simulink model "QArm_Workspace"  (R2022b)
settings: Solver=ode4  StartTime=0.0  StopTime=inf  FixedStep=1/1000  RelTol=1e-3  EnableMultiTasking=on
model workspace (MAT data in the model file):
  cameraStepSize = Simulink.Parameter
  cameraStepSize.Value = Simulink.data.Expression
  cameraStepSize.Value.ExpressionString = "qc_get_step_size * ceil (1/30 /qc_get_step_size)"
  cameraStepSize.DataType = 'auto'
  cameraStepSize.Complexity = 'real'
  cameraStepSize.Dimensions = -1
  mainStepSize = Simulink.Parameter
  mainStepSize.Value = Simulink.data.Expression
  mainStepSize.Value.ExpressionString = "qc_get_step_size"
  mainStepSize.DataType = 'auto'
  mainStepSize.Complexity = 'real'
  mainStepSize.Dimensions = -1
undefined symbols (not defined in the file or in its folder): interleaved, RGB
libraries: quarc_library x14, simulink x2
(part 1 of 2)
settings Model: SimulationMode=external  ExtModeTrigDuration=10000  Creator=mbohra  LastModifiedBy=mbohra
settings SolverCC: AlgebraicLoopSolver=TrustRegion  PositivePriorityOrder=on
settings DataIOCC: ReturnWorkspaceOutputs=off
settings DebuggingCC: UnconnectedInputMsg=warning  UnconnectedOutputMsg=warning  UnconnectedLineMsg=warning  SFMachineParentedDataDiag=warning  ArithmeticOperatorsInVariantConditions=warning
settings ModelReferenceCC: EnableRefExpFcnMdlSchedulingChecks=on
settings SFSimCC: SimUseLocalCustomCode=off  CustomCodeUndefinedFunction=UseInterfaceOnly
settings RTWCC: Description=QUARC Win64 Target Using Toolchain  SystemTargetFile=quarc_win64.tlc  TemplateMakefile=quarc_default_tmf  RTWUseLocalCustomCode=off  Toolchain=QUARC win64 | nmake (64-bit Windows)  BuildConfiguration=Faster Runs  DLArmComputeVersion=19.05
settings CodeAppCC: StateflowObjectComments=on
settings STFCustomTargetCC: TargetLangStandard=C99 (ISO)  ConcurrentExecutionCompliant=on  GRTInterface=on  UseToolchainInfoCompliant=on  SystemTargetFile=quarc_win64.tlc
settings GRTTargetCC: ParMdlRefBuildCompliant=off  CompOptLevelCompliant=off  CombineOutputUpdateFcns=off  MatFileLogging=off  CPPClassGenCompliant=off  GRTInterface=on  ExtMode=on  ExtModeMexFile=quarc_comm
settings ConfigComp: CovMetricSettings=dswe

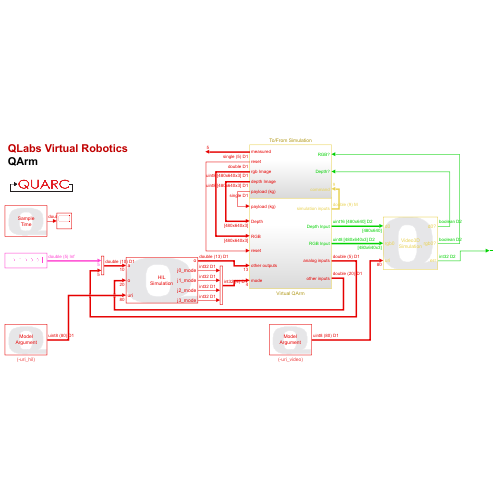
[thumbnail: Simulink's stored preview of the top-level diagram]
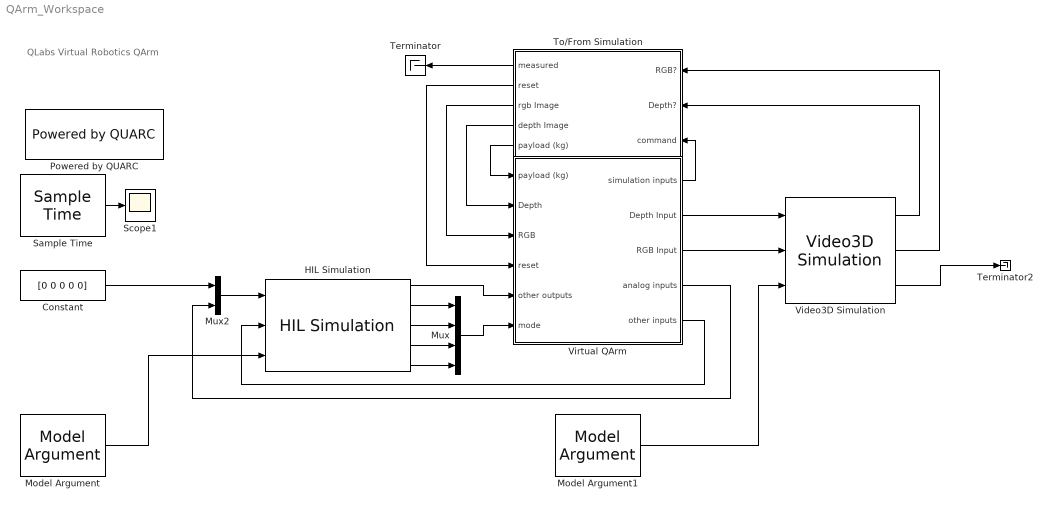
== system QArm_Workspace ==
  note: QLabs Virtual Robotics
      | QArm
  Constant : Constant  Value=[0 0 0 0 0]
  HIL Simulation : quarc_library/Data Acquisition/Generic/Configuration/HIL Simulation  uri_source=External input port  uri=tcpip://localhost:18900  board_type=qarm_usb  board_id=0  options=j0_mode=%d;j1_mode=%d;j2_mode=%d;j3_mode=%d  sample_time=qc_get_step_size  active=on  num_clocks=1  num_interrupts=0  num_analog_inputs=10  num_analog_outputs=0  initial_analog=[]  num_digital_io=0  num_digital_inputs=0  num_digital_outputs=0  initial_digital=[]  num_encoder_inputs=0  num_pwm_outputs=0  initial_pwm=[]  other_inputs=[1000:1004, 3000:3004, 10000:10004, 11000:11004]  other_outputs=[1000:1004, 11000:11003, 11005:11007, 11008]  initial_other=[0 0 0 0 0 0 0 0 0 1 0 0 1]  integer_get_property_codes=[]  double_get_property_codes=[]  string_get_property_codes=[]  integer_set_property_codes=[]  double_set_property_codes=[]  string_set_property_codes=[]  initial_integer_properties=0  initial_double_properties=0  max_string_property=80  use_variable_size_strings=off
      settings: SourceProductName=QUARC Targets
  Model Argument : quarc_library/Sources/Signals/Model Argument  argument_name=uri_hil  has_value=on  data_type_mode=Specify via dialog  data_type=char  max_length=80  default_value=0  default_string=tcpip://localhost:18900  variable_size=off
      settings: AttributesFormatString=(-%<argument_name>)  SourceProductName=QUARC Targets
  Model Argument1 : quarc_library/Sources/Signals/Model Argument  argument_name=uri_video  has_value=on  data_type_mode=Specify via dialog  data_type=char  max_length=80  default_value=0  default_string=tcpip://localhost:18901  variable_size=off
      settings: AttributesFormatString=(-%<argument_name>)  SourceProductName=QUARC Targets
  Mux : Mux
  Mux2 : Mux  Inputs=2
  Powered by QUARC : quarc_library/Logos/Powered by QUARC
  Sample Time : quarc_library/Sources/Time/Sample Time  Priority=-99  sample_time=qc_get_step_size
  Scope1 : Scope
  Terminator : Terminator
  Terminator2 : Terminator
  To/From Simulation : Subsystem
  Video3D Simulation : quarc_library/Multimedia/Video3D Simulation  uri_source=External input port  uri=tcpip://localhost:18901  device_id=0  sample_time=cameraStepSize  show_in_use=on  active=on  depth_indices=[0]  depth_scales=9.44  depth_widths=[640]  depth_heights=[480]  depth_rates=[30]  rgb_indices=[0]  rgb_widths=[640]  rgb_heights=[480]  rgb_rates=[30]  infrared_indices=[]  infrared_widths=[640]  infrared_heights=[480]  infrared_rates=[30]  fisheye_indices=[]  fisheye_widths=[640]  fisheye_heights=[480]  fisheye_rates=[30]  gyro_indices=[]  accel_indices=[]  pose_indices=[]
      settings: SourceProductName=QUARC Targets
  Virtual QArm : Subsystem
  wires:
  Mux2/1 -> HIL Simulation/1
  Constant/1 -> Mux2/1
  HIL Simulation/1 -> Virtual QArm/5(other outputs)
  Virtual QArm/4(analog inputs) -> Mux2/2
  Virtual QArm/5(other inputs) -> HIL Simulation/2
  Virtual QArm/1(simulation inputs) -> To/From Simulation/3(command)
  To/From Simulation/2(reset) -> Virtual QArm/4(reset)
  Sample Time/1 -> Scope1/1
  HIL Simulation/2 -> Mux/1
  HIL Simulation/3 -> Mux/2
  HIL Simulation/4 -> Mux/3
  HIL Simulation/5 -> Mux/4
  Mux/1 -> Virtual QArm/6(mode)
  To/From Simulation/1(measured) -> Terminator/1
  To/From Simulation/4(depth Image) -> Virtual QArm/2("Depth ")
  To/From Simulation/3(rgb Image) -> Virtual QArm/3(RGB)
  Virtual QArm/2(Depth Input) -> Video3D Simulation/1
  Virtual QArm/3(RGB Input) -> Video3D Simulation/2
  Video3D Simulation/3 -> Terminator2/1
  Video3D Simulation/1 -> To/From Simulation/2(Depth?)
  Video3D Simulation/2 -> To/From Simulation/1(RGB?)
  To/From Simulation/5(payload (kg)) -> Virtual QArm/1(payload (kg))
  Model Argument/1 -> HIL Simulation/3
  Model Argument1/1 -> Video3D Simulation/3

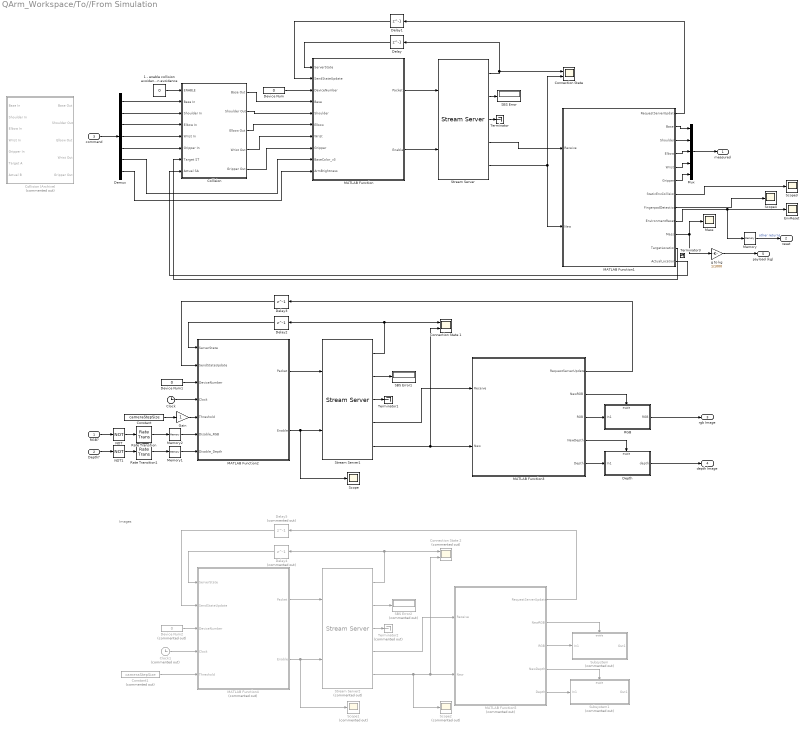
== system QArm_Workspace/To//From Simulation ==
  note: Images
  RGB? : Inport
  Depth? : Inport  Port=2
  command : Inport  Port=3
  1 - enable collision avoidance 0 - disable collision avoidance : Constant  Value=0
  Clock : Clock
  Clock1 : Clock  Commented=on
  Collision : Subsystem
  Collision (Archive) : Subsystem  Commented=on
  "Connection State " : Scope  NumInputPorts=2
  Connection State 1 : Scope  NumInputPorts=2
  Connection State 2 : Scope  Commented=on  NumInputPorts=2
  Constant : Constant  Value=cameraStepSize
  Constant1 : Constant  Commented=on  Value=cameraStepSize
  Delay : Delay  DelayLength=1
  Delay1 : Delay  DelayLength=1
  Delay2 : Delay  DelayLength=1  SampleTime=mainStepSize
  Delay3 : Delay  DelayLength=1  SampleTime=mainStepSize
  Delay4 : Delay  Commented=on  DelayLength=1  SampleTime=mainStepSize
  Delay5 : Delay  Commented=on  DelayLength=1  SampleTime=mainStepSize
  Demux : Demux  Outputs=[1 1 1 1 1 3 1 ]
  Depth : Subsystem
  Device Num : Constant  Value=0
  Device Num1 : Constant  Value=0  SampleTime=mainStepSize
  Device Num2 : Constant  Commented=on  Value=0  SampleTime=mainStepSize
  "EnvReset " : Scope
  Gain : Gain
  MATLAB Function : MATLAB Function  TreatAsAtomicUnit=on
  MATLAB Function1 : MATLAB Function  TreatAsAtomicUnit=on
  MATLAB Function2 : MATLAB Function  TreatAsAtomicUnit=on
  MATLAB Function3 : MATLAB Function  TreatAsAtomicUnit=on
  MATLAB Function4 : MATLAB Function  Commented=on  TreatAsAtomicUnit=on
  MATLAB Function5 : MATLAB Function  Commented=on  TreatAsAtomicUnit=on
  Mass : Scope
  Memory : Memory
  Memory1 : Memory
  Memory2 : Memory
  Mux : Mux  Inputs=5
  NOT : Logic  Operator=NOT  IconShape=distinctive  AllPortsSameDT=off  OutDataTypeStr=boolean
  NOT1 : Logic  Operator=NOT  IconShape=distinctive  AllPortsSameDT=off  OutDataTypeStr=boolean
  RGB : Subsystem
  Rate Transition : RateTransition
  Rate Transition1 : RateTransition
  SBS Error : Display
  SBS Error1 : Display
  SBS Error2 : Display  Commented=on
  Scope : Scope
  Scope1 : Scope  Commented=on
  Scope2 : Scope  Commented=on
  Scope3 : Scope
  Scope4 : Scope
  Stream Server : quarc_library/Communications/Basic/Stream Server  uri_source=Specify via dialog (do not evaluate)  uri=tcpip://remotehost:18001?nagle='off'  send_buffer_size=65537  receive_buffer_size=65537  byte_order=little endian (Intel - LSB first)  optimization=Minimum latency  send_options=Send all data  receive_options=Receive all data  default_value=[0]  sample_time=qc_get_step_size  active=on  implementation=Use blocking I/O in a separate thread  send_fifo_size=3  receive_fifo_size=3  send_priority=0  receive_priority=0  send_dimensions=on  receive_dimensions=on  max_dimensions=65537  data_type=uint8  type_expr=BusObject
      settings: AttributesFormatString="\"tcpip://remotehost:18001?nagle='off'\""
  Stream Server1 : quarc_library/Communications/Basic/Stream Server  uri_source=Specify via dialog (do not evaluate)  uri=tcpip://remotehost:18002?nagle='off'  send_buffer_size=65537  receive_buffer_size=100000  byte_order=little endian (Intel - LSB first)  optimization=Minimum latency  send_options=Send all data  receive_options=Receive all data  default_value=[0]  sample_time=mainStepSize  active=on  implementation=Use blocking I/O in a separate thread  send_fifo_size=3  receive_fifo_size=1  send_priority=0  receive_priority=0  send_dimensions=on  receive_dimensions=on  max_dimensions=65537  data_type=uint8  type_expr=BusObject
      settings: AttributesFormatString="\"tcpip://remotehost:18002?nagle='off'\""
  Stream Server2 : quarc_library/Communications/Basic/Stream Server  Commented=on  uri_source=Specify via dialog (do not evaluate)  uri=tcpip://remotehost:18002?nagle='off'  send_buffer_size=65537  receive_buffer_size=6000000  byte_order=little endian (Intel - LSB first)  optimization=Minimum latency  send_options=Send all data  receive_options=Receive all data  default_value=[0]  sample_time=mainStepSize  active=on  implementation=Use blocking I/O in a separate thread  send_fifo_size=3  receive_fifo_size=1  send_priority=0  receive_priority=0  send_dimensions=on  receive_dimensions=on  max_dimensions=6000000  data_type=uint8  type_expr=BusObject
      settings: AttributesFormatString="\"tcpip://remotehost:18002?nagle='off'\""
  Subsystem : Subsystem  Commented=on
  Subsystem1 : Subsystem  Commented=on
  Terminator : Terminator
  Terminator1 : Terminator
  Terminator2 : Terminator  Commented=on
  Terminator3 : Terminator
  g to kg : Gain  Gain=1/1000
  measured : Outport  VectorParamsAs1DForOutWhenUnconnected=off
  reset : Outport  Port=2  VectorParamsAs1DForOutWhenUnconnected=off
  rgb Image : Outport  Port=3
  depth Image : Outport  Port=4
  payload (kg) : Outport  Port=5
  wires:
  MATLAB Function1/1(RequestServerUpdate) -> Delay1/1
  Mux/1 -> measured/1
  Stream Server/1 -> Delay/1, "Connection State "/1
  Delay1/1 -> MATLAB Function/2(SendStateUpdate)
  Demux/7 -> MATLAB Function/10(ArmBrightness)
  MATLAB Function1/8(FingerpadDetection) -> Scope4/1
  Stream Server/3 -> Terminator/1
  MATLAB Function1/7(StaticEnvCollision) -> Scope3/1
  command/1 -> Demux/1
  Stream Server/2 -> SBS Error/1
  MATLAB Function1/3(Shoulder) -> Mux/2
  Stream Server/5 -> "Connection State "/2, MATLAB Function1/2(New)
  MATLAB Function1/10(Mass) -> Mass/1, g to kg/1
  MATLAB Function/2(Enable) -> Stream Server/2
  Device Num/1 -> MATLAB Function/3(DeviceNumber)
  MATLAB Function/1(Packet) -> Stream Server/1
  Stream Server/4 -> MATLAB Function1/1(Receive)
  MATLAB Function1/6(Gripper) -> Mux/5
  Delay/1 -> MATLAB Function/1(ServerState)
  MATLAB Function1/5(Wrist) -> Mux/4
  MATLAB Function1/4(Elbow) -> Mux/3
  MATLAB Function1/2(Base) -> Mux/1
  Demux/6 -> MATLAB Function/9(BaseColor_v3)
  MATLAB Function1/9(EnvironmentReset) -> Memory/1, "EnvReset "/1
  Memory/1 -> reset/1  "other returns"
  Stream Server1/2 -> SBS Error1/1
  MATLAB Function2/2(Enable) -> Scope/1, Stream Server1/2
  Stream Server1/1 -> Connection State 1/1, Delay2/1
  Clock/1 -> MATLAB Function2/4(Clock)
  MATLAB Function2/1(Packet) -> Stream Server1/1
  Delay2/1 -> MATLAB Function2/1(ServerState)
  Stream Server1/5 -> Connection State 1/2, MATLAB Function3/2(New)
  Stream Server1/3 -> Terminator1/1
  Device Num1/1 -> MATLAB Function2/3(DeviceNumber)
  Delay3/1 -> MATLAB Function2/2(SendStateUpdate)
  Constant/1 -> Gain/1
  Clock1/1 -> MATLAB Function4/4(Clock)
  Delay5/1 -> MATLAB Function4/2(SendStateUpdate)
  Stream Server2/2 -> SBS Error2/1
  MATLAB Function5/1(RequestServerUpdate) -> Delay5/1
  Stream Server2/3 -> Terminator2/1
  Stream Server2/5 -> Scope2/1, Connection State 2/2, MATLAB Function5/2(New)
  MATLAB Function4/1(Packet) -> Stream Server2/1
  Stream Server2/4 -> MATLAB Function5/1(Receive)
  Delay4/1 -> MATLAB Function4/1(ServerState)
  Stream Server2/1 -> Connection State 2/1, Delay4/1
  MATLAB Function4/2(Enable) -> Scope1/1, Stream Server2/2
  Device Num2/1 -> MATLAB Function4/3(DeviceNumber)
  Constant1/1 -> MATLAB Function4/5(Threshold)
  MATLAB Function5/3(RGB) -> Subsystem/1(In1)
  MATLAB Function5/5(Depth) -> Subsystem1/1(In1)
  MATLAB Function5/2(NewRGB) -> Subsystem/Enable
  MATLAB Function5/4(NewDepth) -> Subsystem1/Enable
  Gain/1 -> MATLAB Function2/5(Threshold)
  MATLAB Function3/2(NewRGB) -> RGB/Enable
  MATLAB Function3/5(Depth) -> Depth/1(In1)
  MATLAB Function3/4(NewDepth) -> Depth/Enable
  MATLAB Function3/3(RGB) -> RGB/1(In1)
  MATLAB Function3/1(RequestServerUpdate) -> Delay3/1
  Stream Server1/4 -> MATLAB Function3/1(Receive)
  Depth/1(depth) -> depth Image/1
  RGB/1(RGB) -> rgb Image/1
  Demux/1 -> Collision/2(Base In)
  Demux/2 -> Collision/3(Shoulder In)
  Demux/3 -> Collision/4(Elbow In)
  Demux/4 -> Collision/5(Wrist In)
  Demux/5 -> Collision/6(Gripper In)
  Collision/1("Base Out ") -> MATLAB Function/4(Base)
  Collision/2(Shoulder Out) -> MATLAB Function/5(Shoulder)
  Collision/3(Elbow Out) -> MATLAB Function/6(Elbow)
  Collision/4(Wrist Out) -> MATLAB Function/7(Wrist)
  Collision/5(Gripper Out) -> MATLAB Function/8(Gripper)
  MATLAB Function1/11(TargetLocation) -> Collision/7(Target ST)
  MATLAB Function1/12(ActualLocation) -> Collision/8(Actual SA)
  RGB?/1 -> NOT/1
  Depth?/1 -> NOT1/1
  NOT/1 -> Rate Transition/1
  NOT1/1 -> Rate Transition1/1
  Memory1/1 -> MATLAB Function2/7(Disable_Depth)
  Memory2/1 -> MATLAB Function2/6(Disable_RGB)
  Rate Transition/1 -> Memory2/1
  Rate Transition1/1 -> Memory1/1
  1 - enable collision avoidance 0 - disable collision avoidance/1 -> Collision/1(ENABLE)
  ? -> Terminator3/1
  g to kg/1 -> payload (kg)/1

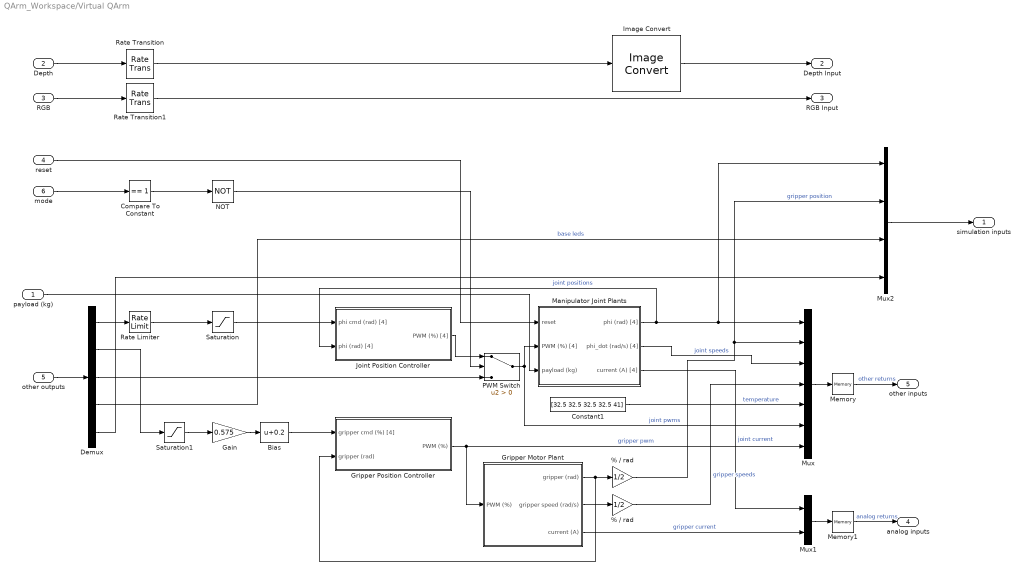
== system QArm_Workspace/Virtual QArm ==
  payload (kg) : Inport
  "Depth " : Inport  Port=2
  RGB : Inport  Port=3
  reset : Inport  Port=4
  other outputs : Inport  Port=5
  mode : Inport  Port=6
  % / rad : Gain  Gain=1/2
  "% / rad " : Gain  Gain=1/2
  Bias : Bias  Bias=0.2  SaturateOnIntegerOverflow=off
  Compare To Constant : simulink/Logic and Bit Operations/Compare To Constant  relop===  const=1  OutDataTypeStr=boolean
  Constant1 : Constant  Value=[32.5 32.5 32.5 32.5 41]
  Demux : Demux  Outputs=[4 1 4 3 1]
  Gain : Gain  Gain=0.575
  Gripper Motor Plant : Subsystem
  Gripper Position Controller : Subsystem
  Image Convert : quarc_library/Image Processing/Generic/Image Convert  input_format=MATLAB RGB (HxWx3)  padding=0  output_format=MATLAB greyscale (HxW)  data_type=uint16
      settings: AttributesFormatString=(%<input_format>)  SourceProductName=QUARC Targets
  Joint Position Controller : Subsystem
  Manipulator Joint Plants : Subsystem
  Memory : Memory  InitialCondition=zeros(1,20)
  Memory1 : Memory  InitialCondition=zeros(1,5)
  Mux : Mux  Inputs=7
  Mux1 : Mux  Inputs=2
  Mux2 : Mux
  NOT : Logic  Operator=NOT  IconShape=distinctive  AllPortsSameDT=off  OutDataTypeStr=boolean
  PWM Switch : Switch  Criteria=u2 > Threshold  SaturateOnIntegerOverflow=off  InputSameDT=off
  Rate Limiter : RateLimiter  RisingSlewLimit=pi/2*[1 1 1 2]  FallingSlewLimit=-pi/2*[1 1 1 2]  SampleTimeMode=inherited
  Rate Transition : RateTransition
  Rate Transition1 : RateTransition
  Saturation : Saturate  UpperLimit=pi*[170 85 75 167.5]/180  LowerLimit=pi*[-170 -85 -95 -167.5]/180
  Saturation1 : Saturate  UpperLimit=1  LowerLimit=0
  simulation inputs : Outport  VectorParamsAs1DForOutWhenUnconnected=off
  Depth Input : Outport  Port=2  VectorParamsAs1DForOutWhenUnconnected=off
  RGB Input : Outport  Port=3  VectorParamsAs1DForOutWhenUnconnected=off
  analog inputs : Outport  Port=4  VectorParamsAs1DForOutWhenUnconnected=off
  other inputs : Outport  Port=5  VectorParamsAs1DForOutWhenUnconnected=off
  wires:
  Gripper Motor Plant/2(gripper speed (rad/s)) -> "% / rad "/1
  PWM Switch/1 -> Mux/6, Manipulator Joint Plants/2(PWM (%) [4])  "joint pwms"
  other outputs/1 -> Demux/1
  Manipulator Joint Plants/1(phi (rad) [4]) -> Mux/1, Mux2/1, Joint Position Controller/2(phi (rad) [4])  "joint positions"
  Demux/3 -> PWM Switch/3
  Mux1/1 -> Memory1/1
  Joint Position Controller/1(PWM (%) [4]) -> PWM Switch/1
  % / rad/1 -> Mux2/2, Mux/2  "gripper position"
  Demux/2 -> Saturation1/1
  Gripper Motor Plant/3(current (A)) -> Mux1/2  "gripper current"
  "% / rad "/1 -> Mux/4  "gripper speeds"
  Gripper Position Controller/1(PWM (%)) -> Mux/7, Gripper Motor Plant/1(PWM (%))  "gripper pwm"
  Gripper Motor Plant/1(gripper (rad)) -> % / rad/1, Gripper Position Controller/2(gripper (rad))
  Saturation1/1 -> Gain/1
  Manipulator Joint Plants/3(current (A) [4]) -> Mux1/1  "joint current"
  Constant1/1 -> Mux/5  "temperature"
  Manipulator Joint Plants/2(phi_dot (rad/s) [4]) -> Mux/3  "joint speeds"
  Demux/1 -> Rate Limiter/1
  Mux/1 -> Memory/1
  Memory/1 -> other inputs/1  "other returns"
  Memory1/1 -> analog inputs/1  "analog returns"
  Mux2/1 -> simulation inputs/1
  mode/1 -> Compare To Constant/1
  Demux/4 -> Mux2/3  "base leds"
  reset/1 -> Manipulator Joint Plants/1(reset)
  Rate Limiter/1 -> Saturation/1
  Compare To Constant/1 -> NOT/1
  NOT/1 -> PWM Switch/2
  Saturation/1 -> Joint Position Controller/1(phi cmd (rad) [4])
  Rate Transition1/1 -> RGB Input/1
  Rate Transition/1 -> Image Convert/1
  "Depth "/1 -> Rate Transition/1
  RGB/1 -> Rate Transition1/1
  Image Convert/1 -> Depth Input/1
  Demux/5 -> Mux2/4
  Bias/1 -> Gripper Position Controller/1(gripper cmd (%) [4])
  Gain/1 -> Bias/1
  payload (kg)/1 -> Manipulator Joint Plants/3(payload (kg))

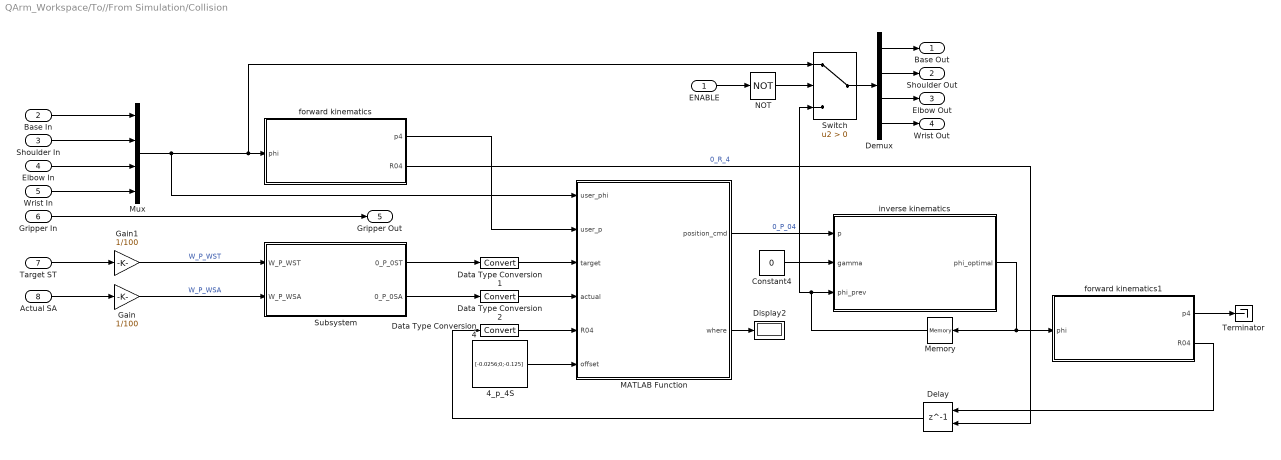
== system QArm_Workspace/To//From Simulation/Collision ==
  ENABLE : Inport
  Base In : Inport  Port=2
  Shoulder In : Inport  Port=3
  Elbow In : Inport  Port=4
  Wrist In : Inport  Port=5
  Gripper In : Inport  Port=6
  Target ST : Inport  Port=7
  Actual SA : Inport  Port=8
  4_p_4S : Constant  Value=[-0.0256;0;-0.125]  VectorParams1D=off
  Constant4 : Constant  Value=0
  Data Type Conversion1 : DataTypeConversion  SaturateOnIntegerOverflow=off  RndMeth=Floor
  Data Type Conversion2 : DataTypeConversion  SaturateOnIntegerOverflow=off  RndMeth=Floor
  Data Type Conversion4 : DataTypeConversion  SaturateOnIntegerOverflow=off  RndMeth=Floor
  Delay : Delay  DelayLength=1  InitialConditionSource=Input port
      settings: InputPortMap=u0,p4
  Demux : Demux
  Display2 : Display
  Gain : Gain  Gain=1/100
  Gain1 : Gain  Gain=1/100
  MATLAB Function : MATLAB Function  TreatAsAtomicUnit=on
  Memory : Memory  InitialCondition=[0 0 0 0]  InheritSampleTime=on
  Mux : Mux
  NOT : Logic  Operator=NOT  IconShape=distinctive  AllPortsSameDT=off  OutDataTypeStr=boolean
  Subsystem : Subsystem
  Switch : Switch  Criteria=u2 > Threshold  SaturateOnIntegerOverflow=off  InputSameDT=off
  Terminator : Terminator
  forward kinematics : MATLAB Function  TreatAsAtomicUnit=on
  forward kinematics1 : MATLAB Function  TreatAsAtomicUnit=on
  inverse kinematics : MATLAB Function  TreatAsAtomicUnit=on
  "Base Out " : Outport  VectorParamsAs1DForOutWhenUnconnected=off
  Shoulder Out : Outport  Port=2  VectorParamsAs1DForOutWhenUnconnected=off
  Elbow Out : Outport  Port=3  VectorParamsAs1DForOutWhenUnconnected=off
  Wrist Out : Outport  Port=4  VectorParamsAs1DForOutWhenUnconnected=off
  Gripper Out : Outport  Port=5  VectorParamsAs1DForOutWhenUnconnected=off
  wires:
  Base In/1 -> Mux/1
  Elbow In/1 -> Mux/3
  Wrist In/1 -> Mux/4
  Gripper In/1 -> Gripper Out/1
  Shoulder In/1 -> Mux/2
  Target ST/1 -> Gain1/1
  Actual SA/1 -> Gain/1
  Gain/1 -> Subsystem/2(W_P_WSA)  "W_P_WSA"
  Gain1/1 -> Subsystem/1(W_P_WST)  "W_P_WST"
  Demux/1 -> "Base Out "/1
  Demux/2 -> Shoulder Out/1
  Demux/3 -> Elbow Out/1
  Demux/4 -> Wrist Out/1
  Switch/1 -> Demux/1
  forward kinematics/2(R04) -> Delay/2  "0_R_4"
  MATLAB Function/1(position_cmd) -> inverse kinematics/1(p)  "0_P_04"
  Delay/1 -> Data Type Conversion4/1
  forward kinematics1/2(R04) -> Delay/1
  inverse kinematics/1(phi_optimal) -> forward kinematics1/1(phi), Memory/1
  Constant4/1 -> inverse kinematics/2(gamma)
  Memory/1 -> Switch/3, inverse kinematics/3(phi_prev)
  Subsystem/2(0_P_0SA) -> Data Type Conversion2/1
  Subsystem/1(0_P_0ST) -> Data Type Conversion1/1
  Mux/1 -> MATLAB Function/1(user_phi), Switch/1, forward kinematics/1(phi)
  forward kinematics/1(p4) -> MATLAB Function/2(user_p)
  Data Type Conversion1/1 -> MATLAB Function/3(target)
  Data Type Conversion2/1 -> MATLAB Function/4(actual)
  Data Type Conversion4/1 -> MATLAB Function/5(R04)
  MATLAB Function/2(where) -> Display2/1
  4_p_4S/1 -> MATLAB Function/6(offset)
  forward kinematics1/1(p4) -> Terminator/1
  ENABLE/1 -> NOT/1
  NOT/1 -> Switch/2

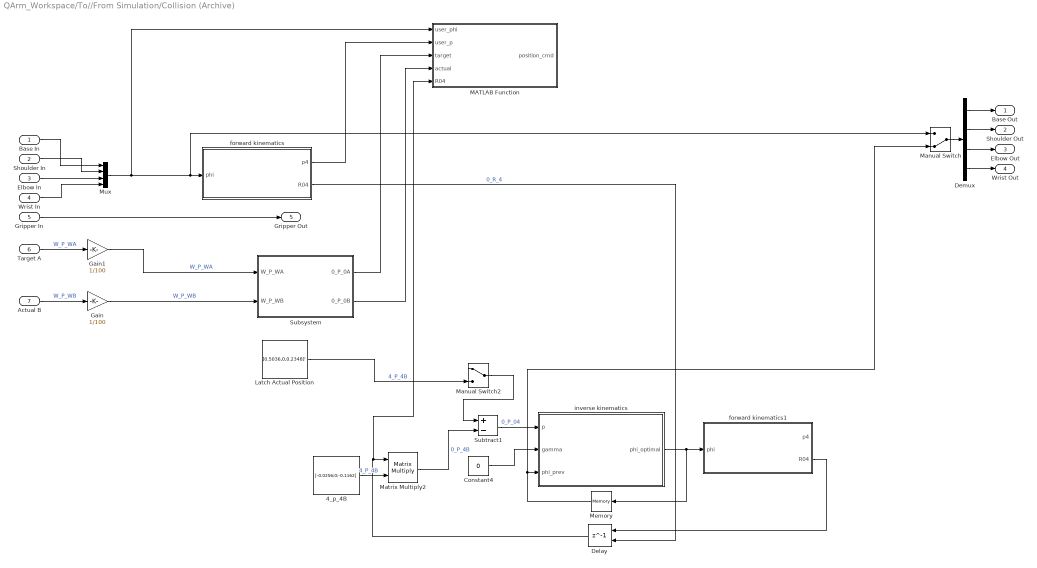
== system QArm_Workspace/To//From Simulation/Collision (Archive) ==
  Base In : Inport
  Shoulder In : Inport  Port=2
  Elbow In : Inport  Port=3
  Wrist In : Inport  Port=4
  Gripper In : Inport  Port=5
  Target A : Inport  Port=6
  Actual B : Inport  Port=7
  4_p_4B : Constant  Value=[-0.0256;0;-0.1162]  VectorParams1D=off
  Constant4 : Constant  Value=0
  Delay : Delay  DelayLength=1  InitialConditionSource=Input port
      settings: InputPortMap=u0,p4
  Demux : Demux
  Gain : Gain  Gain=1/100
  Gain1 : Gain  Gain=1/100
  "Latch Actual Position " : Constant  Value=[0.5036,0,0.2348]'  VectorParams1D=off
  MATLAB Function : MATLAB Function  TreatAsAtomicUnit=on
  Manual Switch : ManualSwitch  CurrentSetting=0
  Manual Switch2 : ManualSwitch
  Matrix Multiply2 : Product  Multiplication=Matrix(*)
  Memory : Memory  InitialCondition=[0 0 0 0]  InheritSampleTime=on
  Mux : Mux
  Subsystem : Subsystem
  Subtract1 : Sum  Inputs=+-
  forward kinematics : MATLAB Function  TreatAsAtomicUnit=on
  forward kinematics1 : MATLAB Function  TreatAsAtomicUnit=on
  inverse kinematics : MATLAB Function  TreatAsAtomicUnit=on
  "Base Out " : Outport  VectorParamsAs1DForOutWhenUnconnected=off
  Shoulder Out : Outport  Port=2  VectorParamsAs1DForOutWhenUnconnected=off
  Elbow Out : Outport  Port=3  VectorParamsAs1DForOutWhenUnconnected=off
  Wrist Out : Outport  Port=4  VectorParamsAs1DForOutWhenUnconnected=off
  Gripper Out : Outport  Port=5  VectorParamsAs1DForOutWhenUnconnected=off
  wires:
  ? -> Manual Switch2/1
  forward kinematics/1(p4) -> MATLAB Function/2(user_p)
  Subsystem/1(0_P_0A) -> MATLAB Function/3(target)
  Subsystem/2(0_P_0B) -> MATLAB Function/4(actual)
  "Latch Actual Position "/1 -> Manual Switch2/2  "4_P_4B"
  Manual Switch2/1 -> Subtract1/1
  Memory/1 -> inverse kinematics/3(phi_prev), Manual Switch/2
  Constant4/1 -> inverse kinematics/2(gamma)
  inverse kinematics/1(phi_optimal) -> forward kinematics1/1(phi), Memory/1
  forward kinematics1/2(R04) -> Delay/1
  Delay/1 -> Matrix Multiply2/1, MATLAB Function/5(R04)
  Subtract1/1 -> inverse kinematics/1(p)  "0_P_04"
  Matrix Multiply2/1 -> Subtract1/2  "0_P_4B"
  4_p_4B/1 -> Matrix Multiply2/2  "4_P_4B"
  forward kinematics/2(R04) -> Delay/2  "0_R_4"
  Manual Switch/1 -> Demux/1
  Demux/4 -> Wrist Out/1
  Demux/3 -> Elbow Out/1
  Demux/2 -> Shoulder Out/1
  Demux/1 -> "Base Out "/1
  Mux/1 -> forward kinematics/1(phi), Manual Switch/1, MATLAB Function/1(user_phi)
  Gain1/1 -> Subsystem/1(W_P_WA)  "W_P_WA"
  Gain/1 -> Subsystem/2(W_P_WB)  "W_P_WB"
  Actual B/1 -> Gain/1  "W_P_WB"
  Target A/1 -> Gain1/1  "W_P_WA"
  Shoulder In/1 -> Mux/2
  Gripper In/1 -> Gripper Out/1
  Wrist In/1 -> Mux/4
  Elbow In/1 -> Mux/3
  Base In/1 -> Mux/1

== system QArm_Workspace/To//From Simulation/Depth ==
  In1 : Inport
  Enable : EnablePort
  Image Decompress : quarc_library/Image Processing/Generic/Image Decompress  algorithm=JPEG  resolution=640 x 480  width=640  height=480  output_format=MATLAB RGB (HxWx3)  data_type=uint8
      settings: AttributesFormatString=(%<algorithm>)  SourceProductName=QUARC Targets
  depth : Outport  VectorParamsAs1DForOutWhenUnconnected=off
  wires:
  Image Decompress/1 -> depth/1
  In1/1 -> Image Decompress/1

== system QArm_Workspace/To//From Simulation/RGB ==
  In1 : Inport
  Enable : EnablePort  PropagateVarSize=During execution
  Image Decompress : quarc_library/Image Processing/Generic/Image Decompress  algorithm=JPEG  resolution=640 x 480  width=640  height=480  output_format=MATLAB RGB (HxWx3)  data_type=uint8
      settings: AttributesFormatString=(%<algorithm>)  SourceProductName=QUARC Targets
  RGB : Outport  VectorParamsAs1DForOutWhenUnconnected=off
  wires:
  In1/1 -> Image Decompress/1
  Image Decompress/1 -> RGB/1

== system QArm_Workspace/To//From Simulation/Subsystem ==
  In1 : Inport
  Enable : EnablePort
  Image Convert : quarc_library/Image Processing/Generic/Image Convert  input_format=RGB (interleaved, 3xWxH)  padding=0  output_format=MATLAB RGB (HxWx3)  data_type=uint8
      settings: AttributesFormatString=(%<input_format>)  SourceProductName=QUARC Targets
  Reshape : Reshape  OutputDimensionality=Customize  OutputDimensions=[3,1280,720]
  Out1 : Outport  VectorParamsAs1DForOutWhenUnconnected=off
  wires:
  Reshape/1 -> Image Convert/1
  In1/1 -> Reshape/1
  Image Convert/1 -> Out1/1

== system QArm_Workspace/To//From Simulation/Subsystem1 ==
  In1 : Inport
  Enable : EnablePort
  Image Convert1 : quarc_library/Image Processing/Generic/Image Convert  input_format=RGB (interleaved, 3xWxH)  padding=0  output_format=MATLAB RGB (HxWx3)  data_type=uint8
      settings: AttributesFormatString=(%<input_format>)  SourceProductName=QUARC Targets
  Reshape1 : Reshape  OutputDimensionality=Customize  OutputDimensions=[3,1280,720]
  Out1 : Outport  VectorParamsAs1DForOutWhenUnconnected=off
  wires:
  Reshape1/1 -> Image Convert1/1
  In1/1 -> Reshape1/1
  Image Convert1/1 -> Out1/1

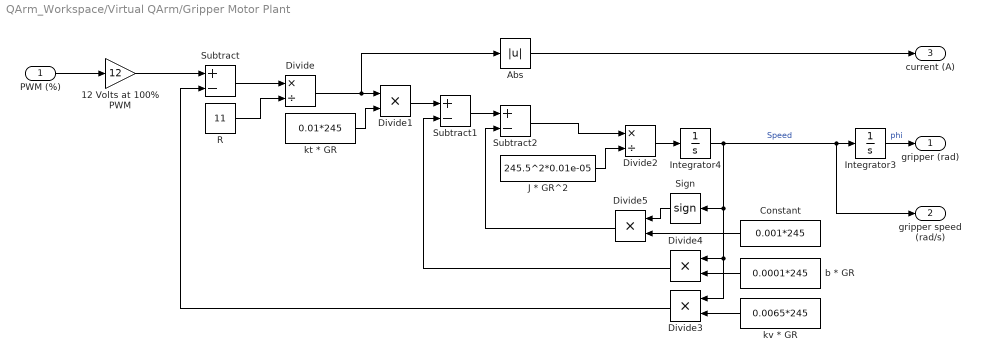
== system QArm_Workspace/Virtual QArm/Gripper Motor Plant ==
  PWM (%) : Inport
  12 Volts at 100% PWM : Gain  Gain=12
  Abs : Abs  SaturateOnIntegerOverflow=off
  Constant : Constant  Value=0.001*245
  Divide : Product  Inputs=*/
  Divide{1,3..5} (4 alike) : Product  Inputs=**
  Divide2 : Product  Inputs=*/
  Integrator3 : Integrator  LimitOutput=on  UpperSaturationLimit=2  LowerSaturationLimit=0
  Integrator4 : Integrator  LimitOutput=on  UpperSaturationLimit=Inf  LowerSaturationLimit=-Inf
  J * GR^2 : Constant  Value=245.5^2*0.01e-05
  R : Constant  Value=11
  Sign : Signum
  Subtract : Sum  Inputs=+-
  Subtract1 : Sum  Inputs=+-
  Subtract2 : Sum  Inputs=+-
  b * GR : Constant  Value=0.0001*245
  kt * GR : Constant  Value=0.01*245
  kv * GR : Constant  Value=0.0065*245
  gripper (rad) : Outport  VectorParamsAs1DForOutWhenUnconnected=off
  gripper speed (rad/s) : Outport  Port=2  VectorParamsAs1DForOutWhenUnconnected=off
  current (A) : Outport  Port=3  VectorParamsAs1DForOutWhenUnconnected=off
  wires:
  Divide4/1 -> Subtract1/2
  Divide2/1 -> Integrator4/1
  Integrator3/1 -> gripper (rad)/1  "phi"
  b * GR/1 -> Divide4/2
  kv * GR/1 -> Divide3/2
  PWM (%)/1 -> 12 Volts at 100% PWM/1
  Subtract1/1 -> Subtract2/1
  J * GR^2/1 -> Divide2/2
  Divide1/1 -> Subtract1/1
  Divide3/1 -> Subtract/2
  Divide/1 -> Divide1/1, Abs/1
  kt * GR/1 -> Divide1/2
  Subtract/1 -> Divide/1
  R/1 -> Divide/2
  Sign/1 -> Divide5/1
  Constant/1 -> Divide5/2
  Integrator4/1 -> Integrator3/1, gripper speed (rad/s)/1, Sign/1, Divide3/1, Divide4/1  "Speed"
  Divide5/1 -> Subtract2/2
  Subtract2/1 -> Divide2/1
  12 Volts at 100% PWM/1 -> Subtract/1
  Abs/1 -> current (A)/1

== system QArm_Workspace/Virtual QArm/Gripper Position Controller ==
  gripper cmd (%) [4] : Inport
  gripper (rad) : Inport  Port=2
  Add : Sum  Inputs=|+-
  Add1 : Sum  Inputs=+++
  Derivative : Derivative
  Gain : Gain  Gain=2048/pi
  Gain1 : Gain  Gain=2048/pi
  Gain2 : Gain  Gain=1/885
  Integrator : Integrator
  Kd : Gain  Gain=0
  Ki : Gain  Gain=0
  Kp : Gain  Gain=700/128
  Saturation : Saturate  UpperLimit=1  LowerLimit=-1
  rad / % : Gain  Gain=2
  PWM (%) : Outport  VectorParamsAs1DForOutWhenUnconnected=off
  wires:
  Kd/1 -> Derivative/1
  Ki/1 -> Integrator/1
  Saturation/1 -> PWM (%)/1
  Derivative/1 -> Add1/3
  Integrator/1 -> Add1/2
  Add/1 -> Kp/1, Ki/1, Kd/1
  Add1/1 -> Gain2/1
  gripper cmd (%) [4]/1 -> rad / %/1
  Kp/1 -> Add1/1
  rad / %/1 -> Gain/1
  gripper (rad)/1 -> Gain1/1
  Gain/1 -> Add/1
  Gain1/1 -> Add/2
  Gain2/1 -> Saturation/1

== system QArm_Workspace/Virtual QArm/Joint Position Controller ==
  phi cmd (rad) [4] : Inport
  phi (rad) [4] : Inport  Port=2
  Add : Sum  Inputs=|+-
  Add1 : Sum  Inputs=+++++
  Derivative : Derivative
  Derivative1 : Derivative
  Derivative2 : Derivative
  Gain : Gain  Gain=2048/pi
  Gain1 : Gain  Gain=2048/pi
  Gain2 : Gain  Gain=1/885
  Gain3 : Gain  Gain=1/4
  Gain4 : Gain  Gain=1/4
  Gain5 : Gain  Gain=1/128
  Gain6 : Gain  Gain=1/65536
  Gain7 : Gain  Gain=1/16
  Integrator : Integrator
  Kd (0 to 16383) : Gain  Gain=[0 0 0 0]
  Kff1 (0 to 16383) : Gain  Gain=[0 0 0 0]
  Kff2 (0 to 16383) : Gain  Gain=[0 0 0 0]
  Ki (0 to 16383) : Gain  Gain=[0 0 0 0]
  Kp (0 to 16383) : Gain  Gain=[800 800 800 800]
  Saturation : Saturate  UpperLimit=[1 1 1 1]  LowerLimit=-1*[1 1 1 1]
  PWM (%) [4] : Outport  VectorParamsAs1DForOutWhenUnconnected=off
  wires:
  phi cmd (rad) [4]/1 -> Gain/1
  phi (rad) [4]/1 -> Gain1/1
  Gain2/1 -> Saturation/1
  Gain1/1 -> Add/2
  Ki (0 to 16383)/1 -> Gain6/1
  Kd (0 to 16383)/1 -> Gain7/1
  Add/1 -> Kd (0 to 16383)/1, Ki (0 to 16383)/1, Kp (0 to 16383)/1
  Integrator/1 -> Add1/4
  Derivative/1 -> Add1/5
  Add1/1 -> Gain2/1
  Gain/1 -> Derivative1/1, Add/1
  Kff2 (0 to 16383)/1 -> Gain4/1
  Derivative1/1 -> Derivative2/1, Kff1 (0 to 16383)/1
  Derivative2/1 -> Kff2 (0 to 16383)/1
  Kff1 (0 to 16383)/1 -> Gain3/1
  Kp (0 to 16383)/1 -> Gain5/1
  Saturation/1 -> PWM (%) [4]/1
  Gain3/1 -> Add1/1
  Gain4/1 -> Add1/2
  Gain5/1 -> Add1/3
  Gain6/1 -> Integrator/1
  Gain7/1 -> Derivative/1

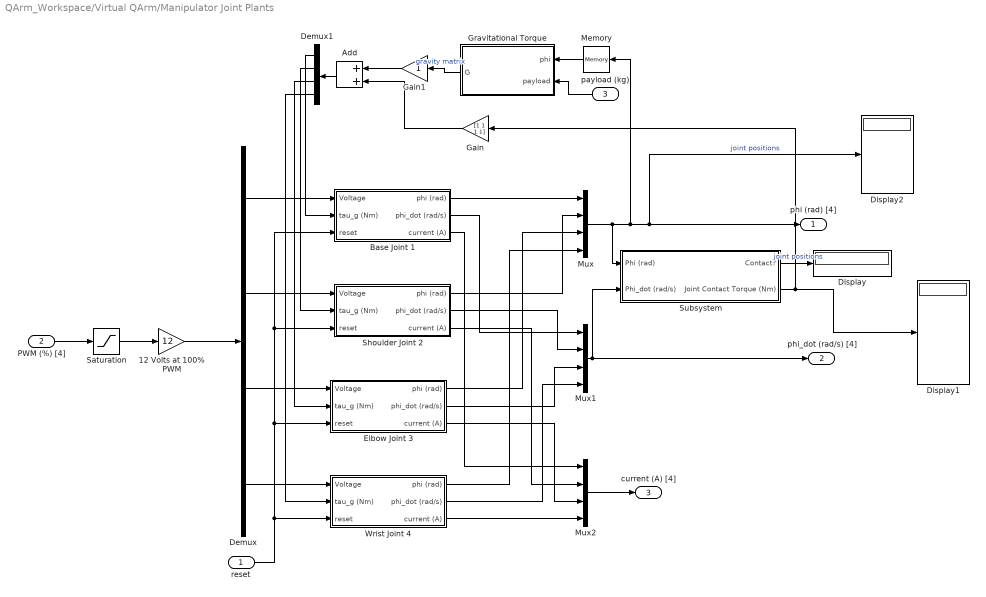
== system QArm_Workspace/Virtual QArm/Manipulator Joint Plants ==
  reset : Inport
  PWM (%) [4] : Inport  Port=2
  payload (kg) : Inport  Port=3
  12 Volts at 100% PWM : Gain  Gain=12
  Add : Sum
  Base Joint 1 : Subsystem
  Demux : Demux
  Demux1 : Demux
  Display : Display
  Display1 : Display
  Display2 : Display
  Elbow Joint 3 : Subsystem
  Gain : Gain  Gain=[1 1 1 1]
  Gain1 : Gain
  Gravitational Torque : MATLAB Function  TreatAsAtomicUnit=on
  Memory : Memory  InitialCondition=[0 0 0 0]
  Mux : Mux
  Mux1 : Mux
  Mux2 : Mux
  Saturation : Saturate  UpperLimit=[1 1 1 1]  LowerLimit=-1*[1 1 1 1]
  Shoulder Joint 2 : Subsystem
  Subsystem : Subsystem
  Wrist Joint 4 : Subsystem
  phi (rad) [4] : Outport  VectorParamsAs1DForOutWhenUnconnected=off
  phi_dot (rad/s) [4] : Outport  Port=2  VectorParamsAs1DForOutWhenUnconnected=off
  current (A) [4] : Outport  Port=3  VectorParamsAs1DForOutWhenUnconnected=off
  wires:
  Mux2/1 -> current (A) [4]/1
  Base Joint 1/1(phi (rad)) -> Mux/1
  Wrist Joint 4/3(current (A)) -> Mux2/4
  Elbow Joint 3/3(current (A)) -> Mux2/3
  Shoulder Joint 2/3(current (A)) -> Mux2/2
  Base Joint 1/3(current (A)) -> Mux2/1
  Wrist Joint 4/2(phi_dot (rad/s)) -> Mux1/4
  Elbow Joint 3/2(phi_dot (rad/s)) -> Mux1/3
  Shoulder Joint 2/2(phi_dot (rad/s)) -> Mux1/2
  Base Joint 1/2(phi_dot (rad/s)) -> Mux1/1
  Wrist Joint 4/1(phi (rad)) -> Mux/4
  Elbow Joint 3/1(phi (rad)) -> Mux/3
  Shoulder Joint 2/1(phi (rad)) -> Mux/2
  12 Volts at 100% PWM/1 -> Demux/1
  Demux/1 -> Base Joint 1/1(Voltage)
  Demux/2 -> Shoulder Joint 2/1(Voltage)
  Demux/3 -> Elbow Joint 3/1(Voltage)
  Demux/4 -> Wrist Joint 4/1(Voltage)
  PWM (%) [4]/1 -> Saturation/1
  Saturation/1 -> 12 Volts at 100% PWM/1
  Memory/1 -> Gravitational Torque/1(phi)
  Gravitational Torque/1(G) -> Gain1/1  "gravity matrix"
  Demux1/1 -> Base Joint 1/2(tau_g (Nm))
  Demux1/2 -> Shoulder Joint 2/2(tau_g (Nm))
  Demux1/3 -> Elbow Joint 3/2(tau_g (Nm))
  Demux1/4 -> Wrist Joint 4/2(tau_g (Nm))
  Add/1 -> Demux1/1
  reset/1 -> Wrist Joint 4/3(reset), Elbow Joint 3/3(reset), Shoulder Joint 2/3(reset), Base Joint 1/3(reset)
  Mux/1 -> Memory/1, Display2/1, phi (rad) [4]/1, Subsystem/1(Phi (rad))  "joint positions"
  Subsystem/1(Contact?) -> Display/1  "joint positions"
  Subsystem/2(Joint Contact Torque (Nm)) -> Display1/1, Gain/1
  Gain/1 -> Add/2
  Gain1/1 -> Add/1
  Mux1/1 -> Subsystem/2(Phi_dot (rad/s)), phi_dot (rad/s) [4]/1
  payload (kg)/1 -> Gravitational Torque/2(payload)

== system QArm_Workspace/To//From Simulation/Collision/Subsystem ==
  W_P_WST : Inport
  W_P_WSA : Inport  Port=2
  0_T_W (Transform from World to Base) : Constant  Value=[0,-1,0,0;-1,0,0,0;0,0,1,0;0,0,0,1]  OutDataTypeStr=single
  Actual Position w.r.t Base : Display
  Constant1 : Constant  OutDataTypeStr=single
  Constant2 : Constant  OutDataTypeStr=single
  Matrix Multiply : Product  Multiplication=Matrix(*)
  Matrix Multiply1 : Product  Multiplication=Matrix(*)
  Mux1 : Mux  Inputs=2
  Mux2 : Mux  Inputs=2
  Reshape : Reshape
  Reshape1 : Reshape
  Selector1 : Selector  InputPortWidth=4  IndexOptions=Index vector (dialog)  Indices=[1:3]  OutputSizes=1
  Selector2 : Selector  InputPortWidth=4  IndexOptions=Index vector (dialog)  Indices=[1:3]  OutputSizes=1
  Target Position w.r.t Base : Display
  0_P_0ST : Outport  VectorParamsAs1DForOutWhenUnconnected=off
  0_P_0SA : Outport  Port=2  VectorParamsAs1DForOutWhenUnconnected=off
  wires:
  Selector1/1 -> 0_P_0SA/1
  0_T_W (Transform from World to Base)/1 -> Matrix Multiply1/1, Matrix Multiply/1  "0_T_W"
  Matrix Multiply1/1 -> Selector1/1, Actual Position w.r.t Base/1  "0_P_0B"
  Reshape/1 -> Matrix Multiply/2
  Constant1/1 -> Mux1/2
  Reshape1/1 -> Matrix Multiply1/2
  Matrix Multiply/1 -> Selector2/1, Target Position w.r.t Base/1  "0_P_0A"
  Mux2/1 -> Reshape1/1
  Mux1/1 -> Reshape/1
  Constant2/1 -> Mux2/2
  W_P_WSA/1 -> Mux2/1
  W_P_WST/1 -> Mux1/1
  Selector2/1 -> 0_P_0ST/1

== system QArm_Workspace/To//From Simulation/Collision (Archive)/Subsystem ==
  W_P_WA : Inport
  W_P_WB : Inport  Port=2
  0_T_W (Transform from World to Base) : Constant  Value=[0,-1,0,0;-1,0,0,0;0,0,1,0;0,0,0,1]  OutDataTypeStr=single
  Actual Position w.r.t Base : Display
  Constant1 : Constant  OutDataTypeStr=single
  Constant2 : Constant  OutDataTypeStr=single
  Matrix Multiply : Product  Multiplication=Matrix(*)
  Matrix Multiply1 : Product  Multiplication=Matrix(*)
  Mux1 : Mux  Inputs=2
  Mux2 : Mux  Inputs=2
  Reshape : Reshape
  Reshape1 : Reshape
  Selector1 : Selector  InputPortWidth=4  IndexOptions=Index vector (dialog)  Indices=[1:3]  OutputSizes=1
  Selector2 : Selector  InputPortWidth=4  IndexOptions=Index vector (dialog)  Indices=[1:3]  OutputSizes=1
  Target Position w.r.t Base : Display
  0_P_0A : Outport  VectorParamsAs1DForOutWhenUnconnected=off
  0_P_0B : Outport  Port=2  VectorParamsAs1DForOutWhenUnconnected=off
  wires:
  Selector2/1 -> 0_P_0A/1
  W_P_WA/1 -> Mux1/1
  W_P_WB/1 -> Mux2/1
  Constant2/1 -> Mux2/2
  Mux1/1 -> Reshape/1
  Mux2/1 -> Reshape1/1
  Matrix Multiply/1 -> Target Position w.r.t Base/1, Selector2/1  "0_P_0A"
  Reshape1/1 -> Matrix Multiply1/2
  Constant1/1 -> Mux1/2
  Reshape/1 -> Matrix Multiply/2
  Matrix Multiply1/1 -> Actual Position w.r.t Base/1, Selector1/1  "0_P_0B"
  0_T_W (Transform from World to Base)/1 -> Matrix Multiply/1, Matrix Multiply1/1  "0_T_W"
  Selector1/1 -> 0_P_0B/1

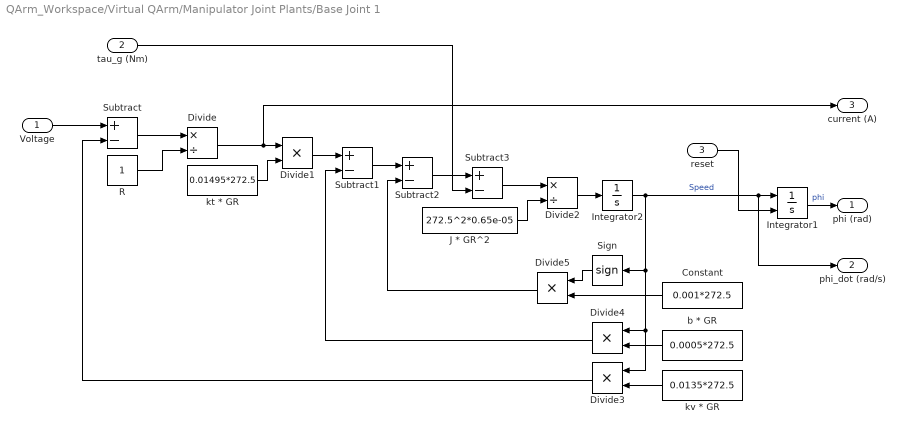
== system QArm_Workspace/Virtual QArm/Manipulator Joint Plants/Base Joint 1 ==
  Voltage : Inport
  tau_g (Nm) : Inport  Port=2
  reset : Inport  Port=3
  Constant : Constant  Value=0.001*272.5
  Divide : Product  Inputs=*/
  Divide{1,3..5} (4 alike) : Product  Inputs=**
  Divide2 : Product  Inputs=*/
  Integrator1 : Integrator  ExternalReset=rising  LimitOutput=on  UpperSaturationLimit=pi*[170]/180  LowerSaturationLimit=pi*[-170]/180
  Integrator2 : Integrator  LimitOutput=on  UpperSaturationLimit=pi/2  LowerSaturationLimit=-pi/2
  J * GR^2 : Constant  Value=272.5^2*0.65e-05
  R : Constant
  Sign : Signum
  Subtract{,1..3} (4 alike) : Sum  Inputs=+-
  b * GR : Constant  Value=0.0005*272.5
  kt * GR : Constant  Value=0.01495*272.5
  kv * GR : Constant  Value=0.0135*272.5
  phi (rad) : Outport  VectorParamsAs1DForOutWhenUnconnected=off
  phi_dot (rad/s) : Outport  Port=2  VectorParamsAs1DForOutWhenUnconnected=off
  current (A) : Outport  Port=3  VectorParamsAs1DForOutWhenUnconnected=off
  wires:
  R/1 -> Divide/2
  Subtract/1 -> Divide/1
  kt * GR/1 -> Divide1/2
  Divide/1 -> current (A)/1, Divide1/1
  Divide3/1 -> Subtract/2
  Divide1/1 -> Subtract1/1
  J * GR^2/1 -> Divide2/2
  Voltage/1 -> Subtract/1
  kv * GR/1 -> Divide3/2
  b * GR/1 -> Divide4/2
  Integrator1/1 -> phi (rad)/1  "phi"
  Divide2/1 -> Integrator2/1
  Divide4/1 -> Subtract1/2
  Constant/1 -> Divide5/2
  Sign/1 -> Divide5/1
  Integrator2/1 -> Sign/1, Divide4/1, Divide3/1, Integrator1/1, phi_dot (rad/s)/1  "Speed"
  Subtract1/1 -> Subtract2/1
  Divide5/1 -> Subtract2/2
  Subtract2/1 -> Subtract3/1
  Subtract3/1 -> Divide2/1
  tau_g (Nm)/1 -> Subtract3/2
  reset/1 -> Integrator1/2

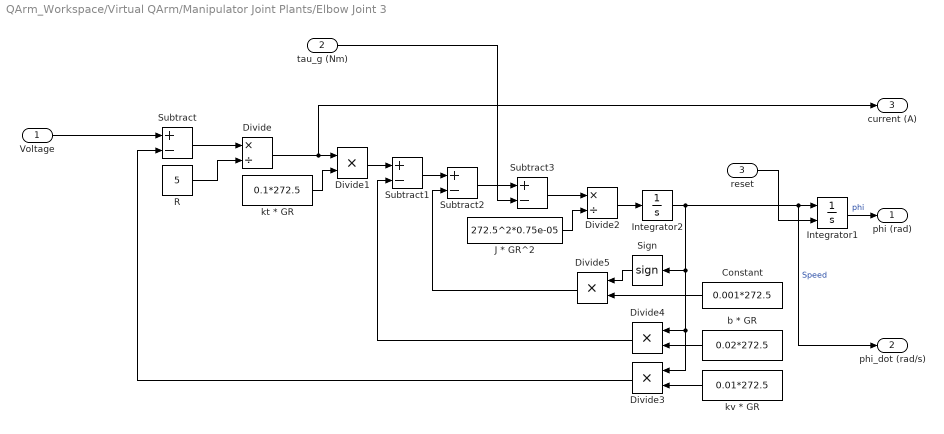
== system QArm_Workspace/Virtual QArm/Manipulator Joint Plants/Elbow Joint 3 ==
  Voltage : Inport
  tau_g (Nm) : Inport  Port=2
  reset : Inport  Port=3
  Constant : Constant  Value=0.001*272.5
  Divide : Product  Inputs=*/
  Divide{1,3..5} (4 alike) : Product  Inputs=**
  Divide2 : Product  Inputs=*/
  Integrator1 : Integrator  ExternalReset=rising  LimitOutput=on  UpperSaturationLimit=pi*[75]/180  LowerSaturationLimit=pi*[-95]/180
  Integrator2 : Integrator  LimitOutput=on  UpperSaturationLimit=pi/2  LowerSaturationLimit=-pi/2
  J * GR^2 : Constant  Value=272.5^2*0.75e-05
  R : Constant  Value=5
  Sign : Signum
  Subtract{,1..3} (4 alike) : Sum  Inputs=+-
  b * GR : Constant  Value=0.02*272.5
  kt * GR : Constant  Value=0.1*272.5
  kv * GR : Constant  Value=0.01*272.5
  phi (rad) : Outport  VectorParamsAs1DForOutWhenUnconnected=off
  phi_dot (rad/s) : Outport  Port=2  VectorParamsAs1DForOutWhenUnconnected=off
  current (A) : Outport  Port=3  VectorParamsAs1DForOutWhenUnconnected=off
  wires:
  R/1 -> Divide/2
  Subtract/1 -> Divide/1
  kt * GR/1 -> Divide1/2
  Divide/1 -> current (A)/1, Divide1/1
  Integrator2/1 -> Divide4/1, Divide3/1, Sign/1, phi_dot (rad/s)/1, Integrator1/1  "Speed"
  Divide3/1 -> Subtract/2
  Divide1/1 -> Subtract1/1
  J * GR^2/1 -> Divide2/2
  Subtract1/1 -> Subtract2/1
  Voltage/1 -> Subtract/1
  kv * GR/1 -> Divide3/2
  b * GR/1 -> Divide4/2
  Integrator1/1 -> phi (rad)/1  "phi"
  Divide2/1 -> Integrator2/1
  Divide4/1 -> Subtract1/2
  Divide5/1 -> Subtract2/2
  Constant/1 -> Divide5/2
  Sign/1 -> Divide5/1
  Subtract3/1 -> Divide2/1
  Subtract2/1 -> Subtract3/1
  tau_g (Nm)/1 -> Subtract3/2
  reset/1 -> Integrator1/2

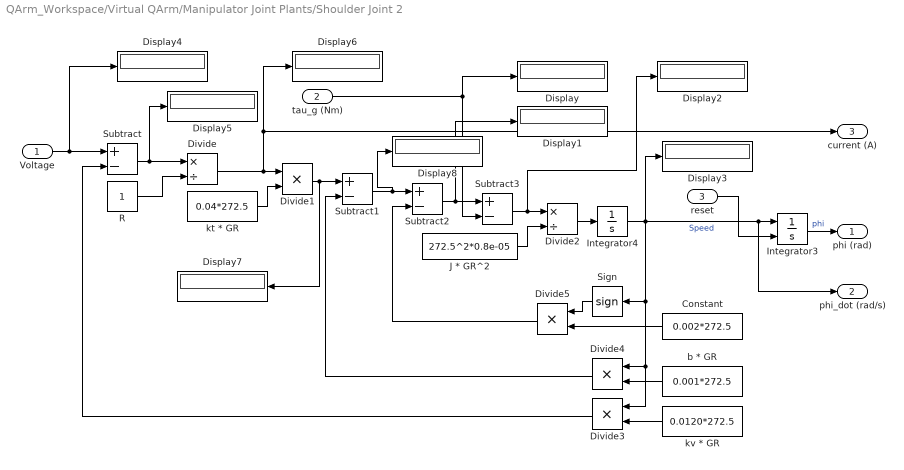
== system QArm_Workspace/Virtual QArm/Manipulator Joint Plants/Shoulder Joint 2 ==
  Voltage : Inport
  tau_g (Nm) : Inport  Port=2
  reset : Inport  Port=3
  Constant : Constant  Value=0.002*272.5
  Display{,1..8} (9 alike) : Display
  Divide : Product  Inputs=*/
  Divide{1,3..5} (4 alike) : Product  Inputs=**
  Divide2 : Product  Inputs=*/
  Integrator3 : Integrator  ExternalReset=rising  LimitOutput=on  UpperSaturationLimit=pi*[85]/180  LowerSaturationLimit=pi*[-85]/180
  Integrator4 : Integrator  LimitOutput=on  UpperSaturationLimit=pi/2  LowerSaturationLimit=-pi/2
  J * GR^2 : Constant  Value=272.5^2*0.8e-05
  R : Constant
  Sign : Signum
  Subtract{,1..3} (4 alike) : Sum  Inputs=+-
  b * GR : Constant  Value=0.001*272.5
  kt * GR : Constant  Value=0.04*272.5
  kv * GR : Constant  Value=0.0120*272.5
  phi (rad) : Outport  VectorParamsAs1DForOutWhenUnconnected=off
  phi_dot (rad/s) : Outport  Port=2  VectorParamsAs1DForOutWhenUnconnected=off
  current (A) : Outport  Port=3  VectorParamsAs1DForOutWhenUnconnected=off
  wires:
  Divide4/1 -> Subtract1/2
  Divide2/1 -> Integrator4/1
  Integrator3/1 -> phi (rad)/1  "phi"
  b * GR/1 -> Divide4/2
  kv * GR/1 -> Divide3/2
  Voltage/1 -> Display4/1, Subtract/1
  Subtract1/1 -> Display8/1, Subtract2/1
  J * GR^2/1 -> Divide2/2
  Divide1/1 -> Subtract1/1, Display7/1
  Divide3/1 -> Subtract/2
  Divide/1 -> Divide1/1, Display6/1, current (A)/1
  kt * GR/1 -> Divide1/2
  Subtract/1 -> Display5/1, Divide/1
  R/1 -> Divide/2
  Constant/1 -> Divide5/2
  Sign/1 -> Divide5/1
  Integrator4/1 -> Display3/1, Integrator3/1, phi_dot (rad/s)/1, Sign/1, Divide3/1, Divide4/1  "Speed"
  Divide5/1 -> Subtract2/2
  Subtract3/1 -> Display2/1, Divide2/1
  Subtract2/1 -> Display1/1, Subtract3/1
  tau_g (Nm)/1 -> Subtract3/2, Display/1
  reset/1 -> Integrator3/2

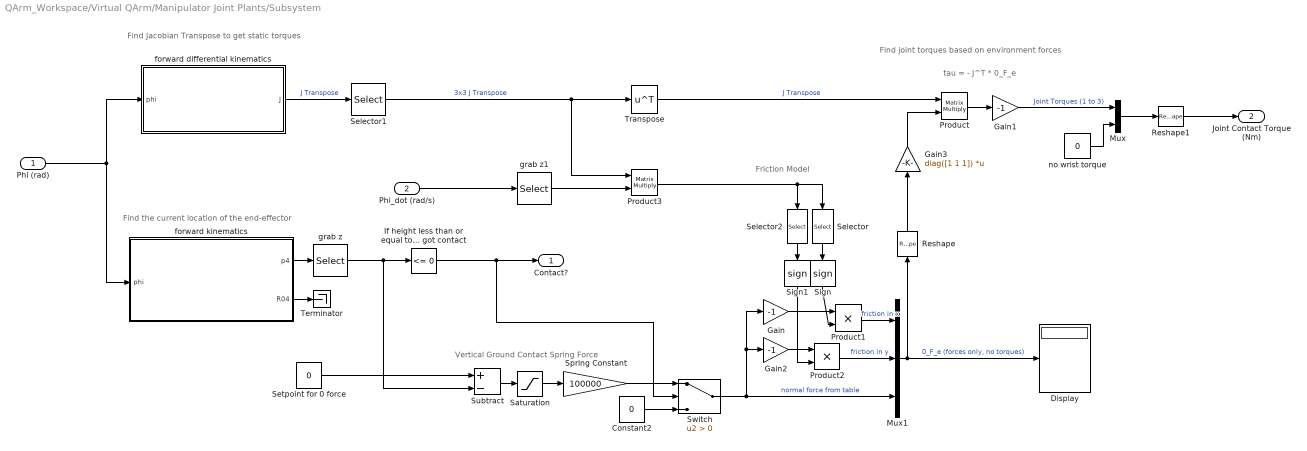
== system QArm_Workspace/Virtual QArm/Manipulator Joint Plants/Subsystem ==
  note: Friction Model
  note: Vertical Ground Contact Spring Force
  note: Find joint torques based on environment forces
  note: Find Jacobian Transpose to get static torques
  note: Find the current location of the end-effector
  note: tau = - J^T * 0_F_e
  Phi (rad) : Inport  PortDimensions=4
  Phi_dot (rad/s) : Inport  Port=2  PortDimensions=4
  Constant2 : Constant  Value=0
  Display : Display
  Gain : Gain  Gain=-1
  Gain1 : Gain  Gain=-1
  Gain2 : Gain  Gain=-1
  Gain3 : Gain  Gain=diag([1 1 1])  Multiplication=Matrix(K*u)
  "If height less than or equal to 0, then we've got contact" : simulink/Logic and Bit Operations/Compare To Constant  relop=<=  const=0  OutDataTypeStr=boolean
  Mux : Mux  Inputs=2
  Mux1 : Mux  Inputs=3
  Product : Product  Multiplication=Matrix(*)
  Product1 : Product
  Product2 : Product
  Product3 : Product  Multiplication=Matrix(*)
  Reshape : Reshape  OutputDimensionality=Column vector (2-D)
  Reshape1 : Reshape
  Saturation : Saturate  UpperLimit=Inf  LowerLimit=0
  Selector : Selector  InputPortWidth=3  IndexOptions=Index vector (dialog)  Indices=1  OutputSizes=1
  Selector1 : Selector  NumberOfDimensions=2  InputPortWidth=3  IndexOptions=Index vector (dialog),Index vector (dialog)  Indices=[1:3],[1:3]  OutputSizes=1,1
  Selector2 : Selector  InputPortWidth=3  IndexOptions=Index vector (dialog)  Indices=2  OutputSizes=1
  Setpoint for 0 force : Constant  Value=0
  Sign : Signum
  Sign1 : Signum
  Spring Constant : Gain  Gain=100000
  Subtract : Sum  Inputs=+-
  Switch : Switch  Criteria=u2 > Threshold  SaturateOnIntegerOverflow=off  InputSameDT=off
  Terminator : Terminator
  Transpose : Math  Operator=transpose  SignedPower=on
  forward differential kinematics : MATLAB Function  TreatAsAtomicUnit=on
  forward kinematics : MATLAB Function  TreatAsAtomicUnit=on
  grab z : Selector  InputPortWidth=3  IndexOptions=Index vector (dialog)  Indices=3  OutputSizes=1
  grab z1 : Selector  InputPortWidth=4  IndexOptions=Index vector (dialog)  Indices=[1:3]  OutputSizes=1
  no wrist torque : Constant  Value=0
  Contact? : Outport  VectorParamsAs1DForOutWhenUnconnected=off
  Joint Contact Torque (Nm) : Outport  Port=2  VectorParamsAs1DForOutWhenUnconnected=off
  wires:
  forward kinematics/1(p4) -> grab z/1
  forward kinematics/2(R04) -> Terminator/1
  grab z/1 -> "If height less than or equal to 0, then we've got contact"/1, Subtract/2
  forward differential kinematics/1(J) -> Selector1/1  "J Transpose"
  Mux1/1 -> Reshape/1, Display/1  "0_F_e (forces only, no torques)"
  Selector1/1 -> Product3/1, Transpose/1  "3x3 J Transpose"
  Product/1 -> Gain1/1
  no wrist torque/1 -> Mux/2
  Mux/1 -> Reshape1/1
  Gain1/1 -> Mux/1  "Joint Torques (1 to 3)"
  Switch/1 -> Mux1/3, Gain2/1, Gain/1  "normal force from table"
  Product2/1 -> Mux1/2  "friction in y"
  "If height less than or equal to 0, then we've got contact"/1 -> Contact?/1, Switch/2
  Constant2/1 -> Switch/3
  Spring Constant/1 -> Switch/1
  Setpoint for 0 force/1 -> Subtract/1
  Subtract/1 -> Saturation/1
  Phi (rad)/1 -> forward differential kinematics/1(phi), forward kinematics/1(phi)
  Reshape/1 -> Gain3/1
  Reshape1/1 -> Joint Contact Torque (Nm)/1
  Product1/1 -> Mux1/1  "friction in x"
  Saturation/1 -> Spring Constant/1
  Phi_dot (rad/s)/1 -> grab z1/1
  Product3/1 -> Selector2/1, Selector/1
  Gain/1 -> Product1/1
  Gain2/1 -> Product2/1
  Selector/1 -> Sign/1
  Selector2/1 -> Sign1/1
  Gain3/1 -> Product/2
  Sign/1 -> Product1/2
  Sign1/1 -> Product2/2
  Transpose/1 -> Product/1  "J Transpose"
  grab z1/1 -> Product3/2

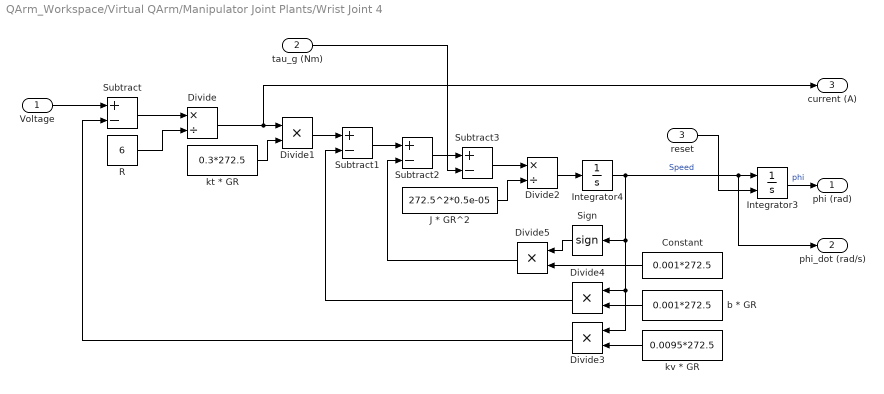
== system QArm_Workspace/Virtual QArm/Manipulator Joint Plants/Wrist Joint 4 ==
  Voltage : Inport
  tau_g (Nm) : Inport  Port=2
  reset : Inport  Port=3
  Constant : Constant  Value=0.001*272.5
  Divide : Product  Inputs=*/
  Divide{1,3..5} (4 alike) : Product  Inputs=**
  Divide2 : Product  Inputs=*/
  Integrator3 : Integrator  ExternalReset=rising  LimitOutput=on  UpperSaturationLimit=pi*[167.5]/180  LowerSaturationLimit=pi*[-167.5]/180
  Integrator4 : Integrator  LimitOutput=on  UpperSaturationLimit=pi  LowerSaturationLimit=-pi
  J * GR^2 : Constant  Value=272.5^2*0.5e-05
  R : Constant  Value=6
  Sign : Signum
  Subtract{,1..3} (4 alike) : Sum  Inputs=+-
  b * GR : Constant  Value=0.001*272.5
  kt * GR : Constant  Value=0.3*272.5
  kv * GR : Constant  Value=0.0095*272.5
  phi (rad) : Outport  VectorParamsAs1DForOutWhenUnconnected=off
  phi_dot (rad/s) : Outport  Port=2  VectorParamsAs1DForOutWhenUnconnected=off
  current (A) : Outport  Port=3  VectorParamsAs1DForOutWhenUnconnected=off
  wires:
  Divide4/1 -> Subtract1/2
  Divide2/1 -> Integrator4/1
  Integrator3/1 -> phi (rad)/1  "phi"
  b * GR/1 -> Divide4/2
  kv * GR/1 -> Divide3/2
  Voltage/1 -> Subtract/1
  Subtract1/1 -> Subtract2/1
  J * GR^2/1 -> Divide2/2
  Divide1/1 -> Subtract1/1
  Divide3/1 -> Subtract/2
  Divide/1 -> Divide1/1, current (A)/1
  kt * GR/1 -> Divide1/2
  Subtract/1 -> Divide/1
  R/1 -> Divide/2
  Sign/1 -> Divide5/1
  Constant/1 -> Divide5/2
  Integrator4/1 -> Integrator3/1, phi_dot (rad/s)/1, Sign/1, Divide3/1, Divide4/1  "Speed"
  Divide5/1 -> Subtract2/2
  Subtract3/1 -> Divide2/1
  Subtract2/1 -> Subtract3/1
  tau_g (Nm)/1 -> Subtract3/2
  reset/1 -> Integrator3/2

== matlab function QArm_Workspace/To//From Simulation/MATLAB Function4 ==
  settings: updateMethod=DISCRETE  sampleTime=mainStepSize
  data: Packet output size=65537; ServerState input; SendStateUpdate input; Enable output; DeviceNumber input; Clock input; Threshold input
function [Packet,Enable] = QArmApplicationWorkspaceMakeVideoPacketData(ServerState, SendStateUpdate, DeviceNumber, Clock, Threshold) 

% Be sure to set the maximum signal size of the variable size Packet port 
% in Simulink->Edit Data of the editor window.  Size should be 65537 or
% larger to ensure that the stream server generates a 4 byte packet size.

%% Setup
persistent LastServerState;
persistent timeLastSend;
persistent readyToSend;

if isempty(LastServerState)
    LastServerState = uint8(0);
    readyToSend = uint8(0);
    timeLastSend = -Threshold;
end

Enable = 0;
Packet = uint8([]);

%% On connection
if ((ServerState == 2) && (LastServerState ~= 2))
    Packet = QArmMakeRGBRawRequestContainer(DeviceNumber);
    Packet = [Packet; QArmMakeDepthRawRequestContainer(DeviceNumber)];
end

%% Send new State Container
% Previous state processed, send a new one
if (SendStateUpdate)
    readyToSend = uint8(1);
end

if readyToSend && ((Clock - timeLastSend) > Threshold)
    Packet = QArmMakeRGBRawRequestContainer(DeviceNumber);
    Packet = [Packet; QArmMakeDepthRawRequestContainer(DeviceNumber)];   
    readyToSend = uint8(0);
    timeLastSend = Clock;
end


%% Transmit
% If we have data to send, enable the transmit
PacketLength = length(Packet);

if (PacketLength > 0)
    % Add magic byte.  This is just for error handling and isn't typically
    % required in simulink, but useful in lower-level languages like Python
    Packet = [uint8(123); Packet];
    
    Enable = 1; 
end

LastServerState = ServerState;

== matlab function QArm_Workspace/Virtual QArm/Manipulator Joint Plants/Gravitational Torque ==
  data: phi input; G output; payload input
function G  = fcn(phi, payload)

%% Manipulator Parameters and Initialization

% Manipulator natural link lengths
L1 = 0.1400;
L2 = 0.3500;
L3 = 0.0500;
L4 = 0.2500;
L5 = 0.1500;

% Manipulator bend angle at joint 3
beta = atan(L3/L2);

% Manipulator mathematical link lenghts
l1 = L1;
l2 = sqrt(L2^2 + L3^2);
l3 = L4 + L5;

% Phi-space to Theta-space
theta = phi;
theta(1) = phi(1);
theta(2) = phi(2) + beta - pi/2;
theta(3) = phi(3) - beta;
theta(4) = phi(4);

%% Dynamic Parameters (Inertias and Masses)

% Masses
mT = 1.75;
m1 = 0.3*mT*l1 / (l1 + l2 + l3);
m2 = mT*l2 / (l1 + l2 + l3);
m3 = mT*L4 / (l1 + l2 + l3);
m4 = mT*L5 / (l1 + l2 + l3);
mL = payload;

% Center of mass locations
% Note: lc1 is unused as the first link does not move linearly (v_1 = 0)
lc2 = l2/2;
lc3 = L4/2;
lc4 = L5/2;

%% Gravity Matrix

g = 9.81;
G2 = -g*(m2*(l2 - lc2)*cos(theta(2)) + m3*(l2*cos(theta(2)) - lc3*sin(theta(2)+theta(3))) + m4*(l2*cos(theta(2)) - (l3 - lc4)*sin(theta(2)+theta(3))) + mL*(l2*cos(theta(2)) - l3*sin(theta(2)+theta(3))) );
G3 = g*(m3*lc3*sin(theta(2)+theta(3)) + m4*(l3 - lc4)*sin(theta(2)+theta(3)) + mL*l3*sin(theta(2)+theta(3)) );

G = [0; G2; G3; 0];
